simulink model "simulation_basic_sil"  (R2022b)
settings: Solver=ode4  StartTime=0.0  StopTime=3  FixedStep=5e-7  MaxStep=1e-6  RelTol=1e-3
undefined symbols (not defined in the file or in its folder): inverter, motor
libraries: eeGeneralControl x6, mcbcontrolslib x5, SignalEditorBlockLib x2, spsTriangleGeneratorLib x1
settings Model: Creator=Rizwan Sadik  LastModifiedBy=Rizwan Sadik

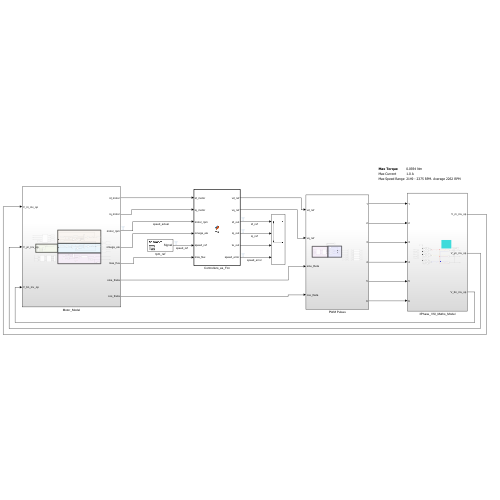
[thumbnail: Simulink's stored preview of the top-level diagram]
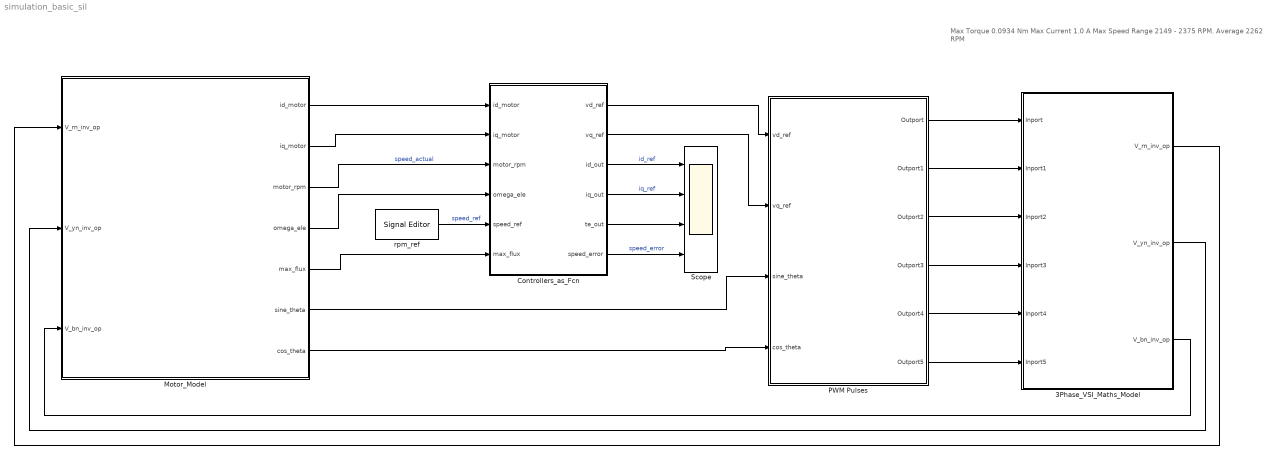
== system simulation_basic_sil ==
  note: Max Torque
      | 0.0934 Nm
      |
      | Max Current
      | 1.0 A
      |
      | Max Speed Range
      | 2149 - 2375 RPM. Average 2262 RPM
  3Phase_VSI_Maths_Model : Subsystem  Description=|
      | Input DC Voltage = Vdc
      | Ouput Phase Voltages = Vrn, Vyn, Vbn
      | 
      | Pole Voltage = Vdc/2
      | Pole Voltages - instantaneous values:
      | Vro = +- Vdc/2
      | Vyo = +- Vdc/2
      | Vbo = +- Vdc/2
      | 
      | Leg 1 o/p is Vr. Switches 1 & 4
      | sw 1 ON (sw 4 OFF) -> Vro = +Vdc/2
      | sw 4 ON (sw 1 OFF) -> Vro = -Vdc/2
      | 
      | Leg 2 o/p is Vy. Switches 3 & 6
      | sw 3 ON (sw 6 OFF) -> Vyo = +Vdc/2
      | sw 6 ON (sw 3 OFF) -> Vyo = -Vdc/2
      | 
      | Leg 3 o/p is Vb. Switches 5 & 2
      | sw 5 ON (sw 2 OFF) -> Vbo = +Vdc/2
      | sw 2 ON (sw 5 OFF) -> Vbo = -Vdc/2
      | 
      | Vrn = (2Vro-Vyo-Vbo)/3
      | Vyn = (2Vyo-Vro-Vbo)/3
      | Vbn =(2Vbo-Vyo-Vro)/3
  Controllers_as_Fcn : MATLAB Function  TreatAsAtomicUnit=on  SystemSampleTime=5e-5
  Motor_Model : Subsystem
  PWM Pulses : Subsystem
  Scope : Scope  NumInputPorts=4
  rpm_ref : SignalEditorBlockLib/Signal Editor  FileName=signal_editor.mat  ActiveScenario=Scenario1  ActiveSignal=Signal  IsBus=off  OutputBusObjectStr=Bus: BusObject  SampleTime=0  ZeroCross=off  OutputAfterFinalValue=Setting to zero  Unit=inherit  PreserveSignalName=on
  wires:
  Motor_Model/3(motor_rpm) -> Controllers_as_Fcn/3(motor_rpm)  "speed_actual"
  Motor_Model/4(omega_ele) -> Controllers_as_Fcn/4(omega_ele)
  PWM Pulses/1(Outport) -> 3Phase_VSI_Maths_Model/1(Inport)
  Motor_Model/5(max_flux) -> Controllers_as_Fcn/6(max_flux)
  PWM Pulses/4(Outport3) -> 3Phase_VSI_Maths_Model/4(Inport3)
  PWM Pulses/5(Outport4) -> 3Phase_VSI_Maths_Model/5(Inport4)
  Motor_Model/6(sine_theta) -> PWM Pulses/3(sine_theta)
  PWM Pulses/3(Outport2) -> 3Phase_VSI_Maths_Model/3(Inport2)
  Motor_Model/2(iq_motor) -> Controllers_as_Fcn/2(iq_motor)
  PWM Pulses/2(Outport1) -> 3Phase_VSI_Maths_Model/2(Inport1)
  PWM Pulses/6(Outport5) -> 3Phase_VSI_Maths_Model/6(Inport5)
  Motor_Model/1(id_motor) -> Controllers_as_Fcn/1(id_motor)
  Motor_Model/7(cos_theta) -> PWM Pulses/4(cos_theta)
  Controllers_as_Fcn/2(vq_ref) -> PWM Pulses/2(vq_ref)
  Controllers_as_Fcn/1(vd_ref) -> PWM Pulses/1(vd_ref)
  3Phase_VSI_Maths_Model/3(V_bn_inv_op) -> Motor_Model/3(V_bn_inv_op)
  3Phase_VSI_Maths_Model/2(V_yn_inv_op) -> Motor_Model/2(V_yn_inv_op)
  3Phase_VSI_Maths_Model/1(V_rn_inv_op) -> Motor_Model/1(V_rn_inv_op)
  rpm_ref/1 -> Controllers_as_Fcn/5(speed_ref)  "speed_ref"
  Controllers_as_Fcn/3(id_out) -> Scope/1  "id_ref"
  Controllers_as_Fcn/4(iq_out) -> Scope/2  "iq_ref"
  Controllers_as_Fcn/5(te_out) -> Scope/3
  Controllers_as_Fcn/6(speed_error) -> Scope/4  "speed_error"

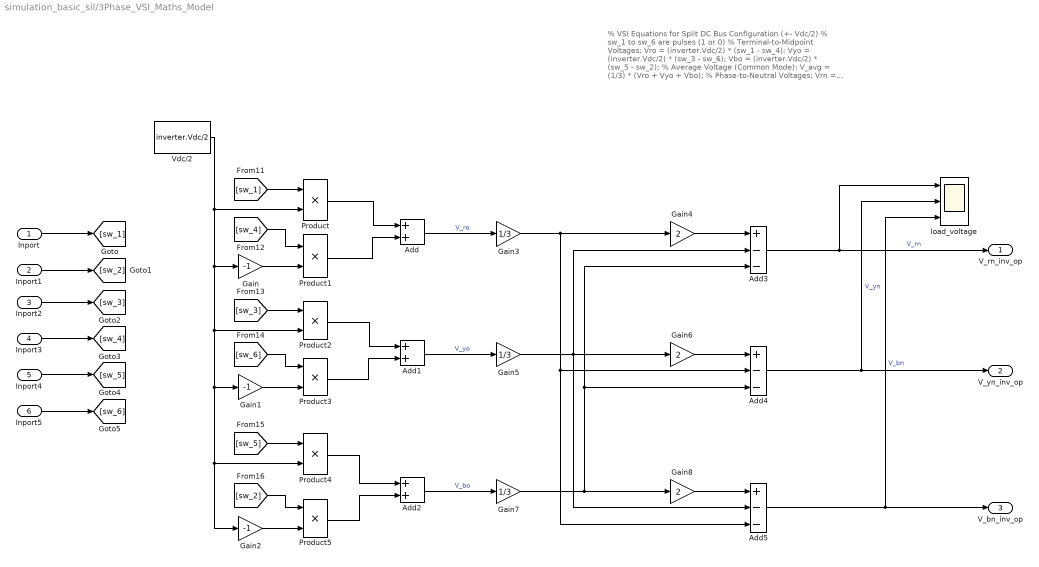
== system simulation_basic_sil/3Phase_VSI_Maths_Model ==
  note: % VSI Equations for Split DC Bus Configuration (+- Vdc/2)
      | % sw_1 to sw_6 are pulses (1 or 0)
      |
      | % Terminal-to-Midpoint Voltages:
      | Vro = (inverter.Vdc/2) * (sw_1 - sw_4);
      | Vyo = (inverter.Vdc/2) * (sw_3 - sw_6);
      | Vbo = (inverter.Vdc/2) * (sw_5 - sw_2);
      |
      | % Average Voltage (Common Mode):
      | V_avg = (1/3) * (Vro + Vyo + Vbo);
      |
      | % Phase-to-Neutral Voltages:
      | Vrn = Vro - V_avg;
      | Vyn = Vyo - V_avg;
      | Vbn = Vbo - V_avg;
  Inport : Inport
  Inport1 : Inport  Port=2
  Inport2 : Inport  Port=3
  Inport3 : Inport  Port=4
  Inport4 : Inport  Port=5
  Inport5 : Inport  Port=6
  Add : Sum
  Add1 : Sum
  Add2 : Sum
  Add3 : Sum  Inputs=+--
  Add4 : Sum  Inputs=+--
  Add5 : Sum  Inputs=+--
  Gain : Gain  Gain=-1
  Gain1 : Gain  Gain=-1
  Gain2 : Gain  Gain=-1
  Gain3 : Gain  Gain=1/3
  Gain4 : Gain  Gain=2
  Gain5 : Gain  Gain=1/3
  Gain6 : Gain  Gain=2
  Gain7 : Gain  Gain=1/3
  Gain8 : Gain  Gain=2
  Product{,1..5} (6 alike) : Product
  Vdc/2 : Constant  Value=inverter.Vdc/2
  load_voltage : Scope  NumInputPorts=3
  V_rn_inv_op : Outport
  V_yn_inv_op : Outport  Port=2
  V_bn_inv_op : Outport  Port=3
  wires:
  Product2/1 -> Add1/1
  Add3/1 -> load_voltage/1, V_rn_inv_op/1  "V_rn"
  Product/1 -> Add/1
  Product4/1 -> Add2/1
  Vdc/2/1 -> Gain2/1, Product4/2, Gain1/1, Product2/2, Gain/1, Product/2
  Gain3/1 -> Add5/3, Add4/2, Gain4/1
  Add4/1 -> load_voltage/2, V_yn_inv_op/1  "V_yn"
  [sw_5] -> Product4/1
  Add/1 -> Gain3/1  "V_ro"
  Gain8/1 -> Add5/1
  Add2/1 -> Gain7/1  "V_bo"
  Gain7/1 -> Gain8/1, Add3/3, Add4/3
  Product5/1 -> Add2/2
  Gain5/1 -> Add5/2, Gain6/1, Add3/2
  [sw_3] -> Product2/1
  Gain4/1 -> Add3/1
  [sw_6] -> Product3/1
  Product3/1 -> Add1/2
  [sw_2] -> Product5/1
  Gain1/1 -> Product3/2
  Gain/1 -> Product1/2
  Product1/1 -> Add/2
  [sw_4] -> Product1/1
  [sw_1] -> Product/1
  Gain2/1 -> Product5/2
  Gain6/1 -> Add4/1
  Add5/1 -> V_bn_inv_op/1, load_voltage/3  "V_bn"
  Inport/1 -> [sw_1]
  Inport1/1 -> [sw_2]
  Inport3/1 -> [sw_4]
  Inport2/1 -> [sw_3]
  Inport5/1 -> [sw_6]
  Inport4/1 -> [sw_5]
  Add1/1 -> Gain5/1  "V_yo"

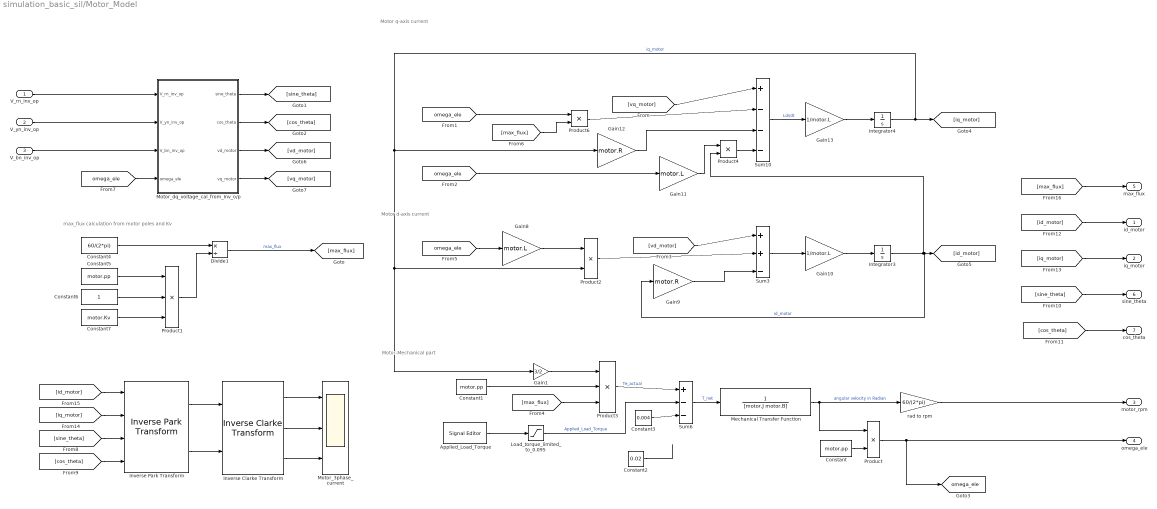
== system simulation_basic_sil/Motor_Model ==
  note: max_flux calculation from motor poles and Kv
  note: Motor-Mechanical part
  note: Motor d-axis current
  note: Motor q-axis current
  V_rn_inv_op : Inport
  V_yn_inv_op : Inport  Port=2
  V_bn_inv_op : Inport  Port=3
  Applied_Load_Torque : SignalEditorBlockLib/Signal Editor  FileName=signal_editor.mat  ActiveScenario=Scenario  ActiveSignal=1  IsBus=off  OutputBusObjectStr=Bus: BusObject  SampleTime=0  ZeroCross=off  OutputAfterFinalValue=Setting to zero  Unit=inherit  PreserveSignalName=on
  Constant : Constant  Value=motor.pp
  Constant1 : Constant  Value=motor.pp
  Constant2 : Constant  Value=0.02
  Constant3 : Constant  Value=0.004
  Constant4 : Constant  Value=60/(2*pi)
  Constant5 : Constant  Value=motor.pp
  Constant6 : Constant
  Constant7 : Constant  Value=motor.Kv
  Divide1 : Product  Inputs=*/
  Gain1 : Gain  Gain=3/2
  Gain10 : Gain  Gain=1/motor.L
  Gain11 : Gain  Gain=motor.L
  Gain12 : Gain  Gain=motor.R
  Gain13 : Gain  Gain=1/motor.L
  Gain8 : Gain  Gain=motor.L
  Gain9 : Gain  Gain=motor.R
  Integrator3 : Integrator
  Integrator4 : Integrator
  Inverse Clarke Transform : mcbcontrolslib/Inverse Clarke Transform
      settings: LibrarySourceBlock=mcbhdllib/Controls/Math Transforms/Inverse Clarke Transform
  Inverse Park Transform : mcbcontrolslib/Inverse Park Transform  AxisAlignment=D-axis
      settings: LibrarySourceBlock=mcblib/Controls/Math Transforms/Inverse Park Transform
  Load_torque_limited_to_0.095 : Saturate  UpperLimit=0.095  LowerLimit=0
  Mechanical Transfer Function : TransferFcn  Denominator=[motor.J motor.B]
  Motor_3phase_current : Scope  NumInputPorts=3
  Motor_dq_voltage_cal_from_Inv_o/p : Subsystem
  Product{,2,4,6} (4 alike) : Product
  Product1 : Product  Inputs=3
  Product3 : Product  Inputs=3
  Sum10 : Sum  Inputs=|+---
  Sum3 : Sum  Inputs=|++-
  Sum6 : Sum  Inputs=+|--
  rad to rpm : Gain  Gain=60/(2*pi)
  id_motor : Outport
  iq_motor : Outport  Port=2
  motor_rpm : Outport  Port=3
  omega_ele : Outport  Port=4
  max_flux : Outport  Port=5
  sine_theta : Outport  Port=6
  cos_theta : Outport  Port=7
  tag scope: omega_ele=global
  wires:
  Product6/1 -> Sum10/2
  Gain12/1 -> Sum10/3
  [max_flux] -> Product6/2
  Gain13/1 -> Integrator4/1
  Gain11/1 -> Product4/1
  Integrator4/1 -> [iq_motor], Gain1/1, Product2/2, Gain12/1  "iq_motor"
  Product4/1 -> Sum10/4
  [omega_ele] -> Gain11/1
  Sum10/1 -> Gain13/1  "Ldi/dt​​"
  [vq_motor] -> Sum10/1
  [omega_ele] -> Product6/1
  Product2/1 -> Sum3/2
  Integrator3/1 -> [id_motor], Gain9/1, Product4/2  "id_motor"
  Gain9/1 -> Sum3/3
  Gain8/1 -> Product2/1
  Sum3/1 -> Gain10/1
  Gain10/1 -> Integrator3/1
  [omega_ele] -> Gain8/1
  [vd_motor] -> Sum3/1
  [max_flux] -> Product3/3
  Constant/1 -> Product/2
  Product/1 -> omega_ele/1, [omega_ele]
  Mechanical Transfer Function/1 -> rad to rpm/1, Product/1  "angular velocity in Radian"
  Sum6/1 -> Mechanical Transfer Function/1  "T_net"
  Constant3/1 -> Sum6/3
  Gain1/1 -> Product3/1
  Product3/1 -> Sum6/1  "Te_actual"
  Load_torque_limited_to_0.095/1 -> Sum6/2  "Applied_Load_Torque"
  Constant1/1 -> Product3/2
  rad to rpm/1 -> motor_rpm/1
  Constant6/1 -> Product1/2
  Product1/1 -> Divide1/2
  Constant5/1 -> Product1/1
  Constant7/1 -> Product1/3
  Constant4/1 -> Divide1/1
  Divide1/1 -> [max_flux]  "max_flux"
  Applied_Load_Torque/1 -> Load_torque_limited_to_0.095/1
  V_rn_inv_op/1 -> Motor_dq_voltage_cal_from_Inv_o/p/1(V_rn_inv_op)
  V_yn_inv_op/1 -> Motor_dq_voltage_cal_from_Inv_o/p/2(V_yn_inv_op)
  V_bn_inv_op/1 -> Motor_dq_voltage_cal_from_Inv_o/p/3(V_bn_inv_op)
  [omega_ele] -> Motor_dq_voltage_cal_from_Inv_o/p/4(omega_ele)
  Motor_dq_voltage_cal_from_Inv_o/p/2(cos_theta) -> [cos_theta]
  Motor_dq_voltage_cal_from_Inv_o/p/3(vd_motor) -> [vd_motor]
  Motor_dq_voltage_cal_from_Inv_o/p/4(vq_motor) -> [vq_motor]
  Inverse Clarke Transform/2 -> Motor_3phase_current/2
  Inverse Clarke Transform/1 -> Motor_3phase_current/1
  Inverse Park Transform/1 -> Inverse Clarke Transform/1
  Inverse Clarke Transform/3 -> Motor_3phase_current/3
  Inverse Park Transform/2 -> Inverse Clarke Transform/2
  Motor_dq_voltage_cal_from_Inv_o/p/1(sine_theta) -> [sine_theta]
  [sine_theta] -> Inverse Park Transform/3
  [cos_theta] -> Inverse Park Transform/4
  [sine_theta] -> sine_theta/1
  [cos_theta] -> cos_theta/1
  [id_motor] -> id_motor/1
  [iq_motor] -> iq_motor/1
  [iq_motor] -> Inverse Park Transform/2
  [id_motor] -> Inverse Park Transform/1
  [max_flux] -> max_flux/1
  Constant2/1 -> ?

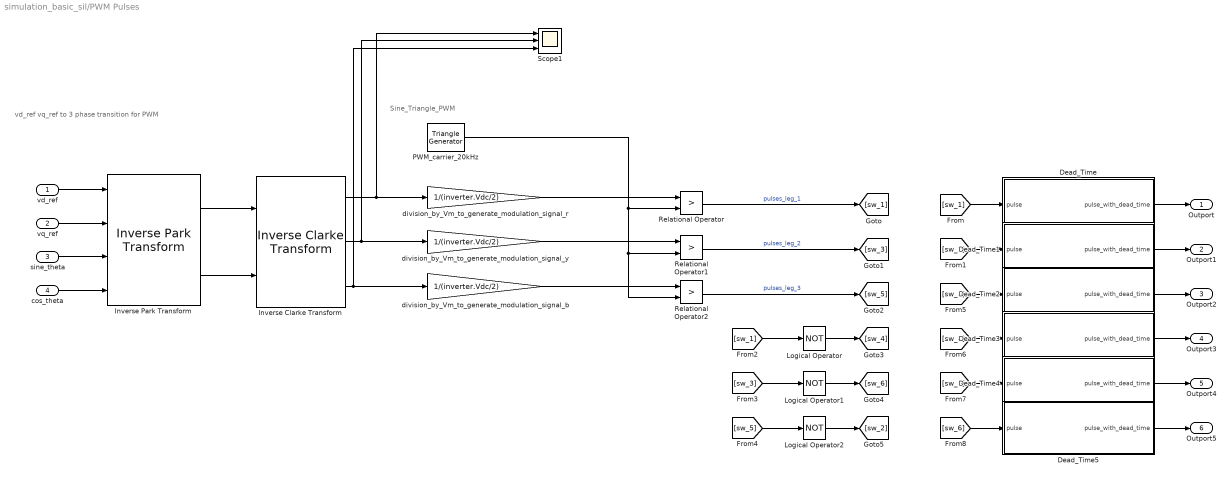
== system simulation_basic_sil/PWM Pulses ==
  note: vd_ref vq_ref to 3 phase transition for PWM
  note: Sine_Triangle_PWM
  vd_ref : Inport
  vq_ref : Inport  Port=2
  sine_theta : Inport  Port=3
  cos_theta : Inport  Port=4
  Dead_Time : Subsystem
  Dead_Time1 : Subsystem
  Dead_Time2 : Subsystem
  Dead_Time3 : Subsystem
  Dead_Time4 : Subsystem
  Dead_Time5 : Subsystem
  Inverse Clarke Transform : mcbcontrolslib/Inverse Clarke Transform
      settings: LibrarySourceBlock=mcbhdllib/Controls/Math Transforms/Inverse Clarke Transform
  Inverse Park Transform : mcbcontrolslib/Inverse Park Transform  AxisAlignment=D-axis
      settings: LibrarySourceBlock=mcblib/Controls/Math Transforms/Inverse Park Transform
  Logical Operator : Logic  Operator=NOT  AllPortsSameDT=off  OutDataTypeStr=boolean
  Logical Operator1 : Logic  Operator=NOT  AllPortsSameDT=off  OutDataTypeStr=boolean
  Logical Operator2 : Logic  Operator=NOT  AllPortsSameDT=off  OutDataTypeStr=boolean
  PWM_carrier_20kHz : spsTriangleGeneratorLib/Triangle Generator  Freq=20000  Phase=0  Ts=0
  Relational Operator : RelationalOperator  Operator=>  OutDataTypeStr=boolean  RndMeth=Simplest  InputSameDT=off
  Relational Operator1 : RelationalOperator  Operator=>  OutDataTypeStr=boolean  RndMeth=Simplest  InputSameDT=off
  Relational Operator2 : RelationalOperator  Operator=>  OutDataTypeStr=boolean  RndMeth=Simplest  InputSameDT=off
  Scope1 : Scope  NumInputPorts=3
  division_by_Vm_to_generate_modulation_signal_b : Gain  Gain=1/(inverter.Vdc/2)
  division_by_Vm_to_generate_modulation_signal_r : Gain  Gain=1/(inverter.Vdc/2)
  division_by_Vm_to_generate_modulation_signal_y : Gain  Gain=1/(inverter.Vdc/2)
  Outport : Outport
  Outport1 : Outport  Port=2
  Outport2 : Outport  Port=3
  Outport3 : Outport  Port=4
  Outport4 : Outport  Port=5
  Outport5 : Outport  Port=6
  wires:
  [sw_3] -> Logical Operator1/1
  Logical Operator2/1 -> [sw_2]
  cos_theta/1 -> Inverse Park Transform/4
  sine_theta/1 -> Inverse Park Transform/3
  [sw_5] -> Logical Operator2/1
  Inverse Park Transform/2 -> Inverse Clarke Transform/2
  Inverse Park Transform/1 -> Inverse Clarke Transform/1
  Logical Operator/1 -> [sw_4]
  Logical Operator1/1 -> [sw_6]
  [sw_1] -> Logical Operator/1
  vd_ref/1 -> Inverse Park Transform/1
  vq_ref/1 -> Inverse Park Transform/2
  [sw_1] -> Dead_Time/1(pulse)
  [sw_6] -> Dead_Time5/1(pulse)
  [sw_2] -> Dead_Time1/1(pulse)
  [sw_3] -> Dead_Time2/1(pulse)
  [sw_4] -> Dead_Time3/1(pulse)
  [sw_5] -> Dead_Time4/1(pulse)
  Relational Operator2/1 -> [sw_5]  "pulses_leg_3"
  Relational Operator1/1 -> [sw_3]  "pulses_leg_2"
  Relational Operator/1 -> [sw_1]  "pulses_leg_1"
  PWM_carrier_20kHz/1 -> Relational Operator2/2, Relational Operator1/2, Relational Operator/2
  division_by_Vm_to_generate_modulation_signal_y/1 -> Relational Operator1/1
  division_by_Vm_to_generate_modulation_signal_b/1 -> Relational Operator2/1
  Inverse Clarke Transform/3 -> Scope1/3, division_by_Vm_to_generate_modulation_signal_b/1
  Inverse Clarke Transform/2 -> Scope1/2, division_by_Vm_to_generate_modulation_signal_y/1
  division_by_Vm_to_generate_modulation_signal_r/1 -> Relational Operator/1
  Inverse Clarke Transform/1 -> Scope1/1, division_by_Vm_to_generate_modulation_signal_r/1
  Dead_Time/1(pulse_with_dead_time) -> Outport/1
  Dead_Time1/1(pulse_with_dead_time) -> Outport1/1
  Dead_Time2/1(pulse_with_dead_time) -> Outport2/1
  Dead_Time3/1(pulse_with_dead_time) -> Outport3/1
  Dead_Time4/1(pulse_with_dead_time) -> Outport4/1
  Dead_Time5/1(pulse_with_dead_time) -> Outport5/1

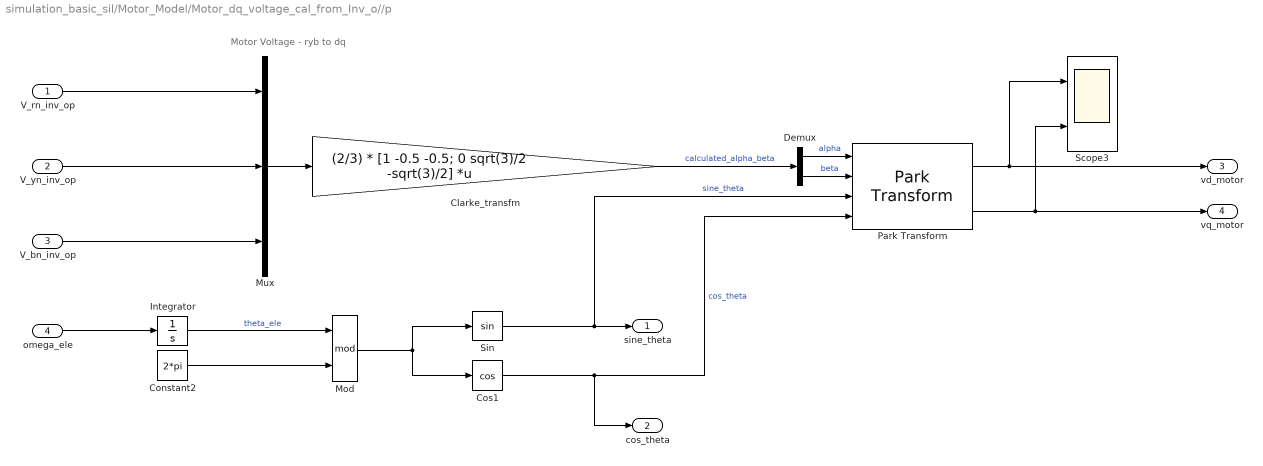
== system simulation_basic_sil/Motor_Model/Motor_dq_voltage_cal_from_Inv_o//p ==
  note: Motor Voltage - ryb to dq
  V_rn_inv_op : Inport
  V_yn_inv_op : Inport  Port=2
  V_bn_inv_op : Inport  Port=3
  omega_ele : Inport  Port=4
  Clarke_transfm : Gain  Gain=(2/3) * [1 -0.5 -0.5; 0 sqrt(3)/2 -sqrt(3)/2]  Multiplication=Matrix(K*u)
  Constant2 : Constant  Value=2*pi
  Cos1 : Trigonometry  Operator=cos
  Demux : Demux  Outputs=2
  Integrator : Integrator
  Mod : Math  Operator=mod
  Mux : Mux  Inputs=3
  Park Transform : mcbcontrolslib/Park Transform  AxisAlignment=D-axis
      settings: LibrarySourceBlock=mcbhdllib/Controls/Math Transforms/Park Transform
  Scope3 : Scope  NumInputPorts=2
  Sin : Trigonometry
  sine_theta : Outport
  cos_theta : Outport  Port=2
  vd_motor : Outport  Port=3
  vq_motor : Outport  Port=4
  wires:
  Sin/1 -> sine_theta/1, Park Transform/3  "sine_theta"
  Constant2/1 -> Mod/2
  Cos1/1 -> cos_theta/1, Park Transform/4  "cos_theta"
  Mod/1 -> Cos1/1, Sin/1
  Demux/1 -> Park Transform/1  "alpha"
  Park Transform/2 -> Scope3/2, vq_motor/1
  Clarke_transfm/1 -> Demux/1  "calculated_alpha_beta"
  Integrator/1 -> Mod/1  "theta_ele"
  Demux/2 -> Park Transform/2  "beta"
  Mux/1 -> Clarke_transfm/1
  Park Transform/1 -> vd_motor/1, Scope3/1
  V_bn_inv_op/1 -> Mux/3
  omega_ele/1 -> Integrator/1
  V_rn_inv_op/1 -> Mux/1
  V_yn_inv_op/1 -> Mux/2

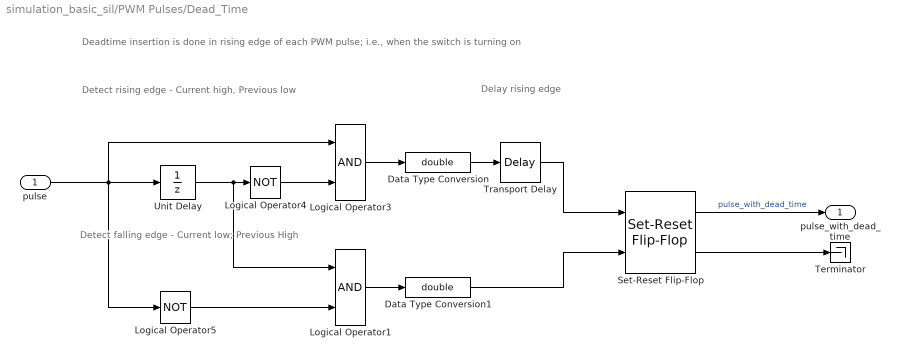
== system simulation_basic_sil/PWM Pulses/Dead_Time ==
  note: Deadtime insertion is done in rising edge of each PWM pulse; i.e., when the switch is turning on
  note: Delay rising edge
  note: Detect falling edge - Current low; Previous High
  note: Detect rising edge - Current high, Previous low
  pulse : Inport
  Data Type Conversion : DataTypeConversion  OutDataTypeStr=double  SaturateOnIntegerOverflow=off  RndMeth=Floor
  Data Type Conversion1 : DataTypeConversion  OutDataTypeStr=double  SaturateOnIntegerOverflow=off  RndMeth=Floor
  Logical Operator1 : Logic  AllPortsSameDT=off  OutDataTypeStr=boolean
  Logical Operator3 : Logic  AllPortsSameDT=off  OutDataTypeStr=boolean
  Logical Operator4 : Logic  Operator=NOT  AllPortsSameDT=off  OutDataTypeStr=boolean
  Logical Operator5 : Logic  Operator=NOT  AllPortsSameDT=off  OutDataTypeStr=boolean
  Set-Reset Flip-Flop : eeGeneralControl/Set-Reset Flip-Flop  LabelModeActiveChoice=Discrete  UndefState=Set  Q0=0  Ts=-1
      settings: LibrarySourceBlock=ee_sl_lib/General Control/Set-Reset Flip-Flop
  Terminator : Terminator
  Transport Delay : TransportDelay  DelayTime=2e-6
  Unit Delay : UnitDelay  SampleTime=-1  HasFrameUpgradeWarning=on
  pulse_with_dead_time : Outport
  wires:
  Unit Delay/1 -> Logical Operator1/1, Logical Operator4/1
  pulse/1 -> Logical Operator5/1, Logical Operator3/1, Unit Delay/1
  Logical Operator5/1 -> Logical Operator1/2
  Logical Operator4/1 -> Logical Operator3/2
  Transport Delay/1 -> Set-Reset Flip-Flop/1
  Data Type Conversion/1 -> Transport Delay/1
  Logical Operator3/1 -> Data Type Conversion/1
  Data Type Conversion1/1 -> Set-Reset Flip-Flop/2
  Logical Operator1/1 -> Data Type Conversion1/1
  Set-Reset Flip-Flop/1 -> pulse_with_dead_time/1  "pulse_with_dead_time"
  Set-Reset Flip-Flop/2 -> Terminator/1

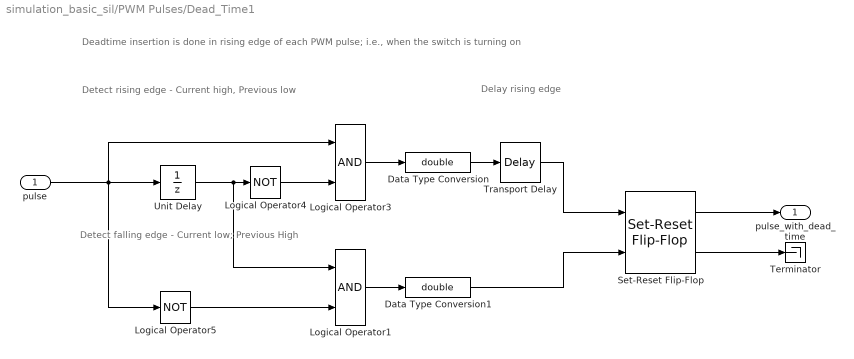
== system simulation_basic_sil/PWM Pulses/Dead_Time1 ==
  note: Detect rising edge - Current high, Previous low
  note: Detect falling edge - Current low; Previous High
  note: Delay rising edge
  note: Deadtime insertion is done in rising edge of each PWM pulse; i.e., when the switch is turning on
  pulse : Inport
  Data Type Conversion : DataTypeConversion  OutDataTypeStr=double  SaturateOnIntegerOverflow=off  RndMeth=Floor
  Data Type Conversion1 : DataTypeConversion  OutDataTypeStr=double  SaturateOnIntegerOverflow=off  RndMeth=Floor
  Logical Operator1 : Logic  AllPortsSameDT=off  OutDataTypeStr=boolean
  Logical Operator3 : Logic  AllPortsSameDT=off  OutDataTypeStr=boolean
  Logical Operator4 : Logic  Operator=NOT  AllPortsSameDT=off  OutDataTypeStr=boolean
  Logical Operator5 : Logic  Operator=NOT  AllPortsSameDT=off  OutDataTypeStr=boolean
  Set-Reset Flip-Flop : eeGeneralControl/Set-Reset Flip-Flop  LabelModeActiveChoice=Discrete  UndefState=Set  Q0=0  Ts=-1
      settings: LibrarySourceBlock=ee_sl_lib/General Control/Set-Reset Flip-Flop
  Terminator : Terminator
  Transport Delay : TransportDelay  DelayTime=2e-6
  Unit Delay : UnitDelay  SampleTime=-1  HasFrameUpgradeWarning=on
  pulse_with_dead_time : Outport
  wires:
  Set-Reset Flip-Flop/2 -> Terminator/1
  Set-Reset Flip-Flop/1 -> pulse_with_dead_time/1
  Logical Operator1/1 -> Data Type Conversion1/1
  Data Type Conversion1/1 -> Set-Reset Flip-Flop/2
  Logical Operator3/1 -> Data Type Conversion/1
  Data Type Conversion/1 -> Transport Delay/1
  Transport Delay/1 -> Set-Reset Flip-Flop/1
  Logical Operator4/1 -> Logical Operator3/2
  Logical Operator5/1 -> Logical Operator1/2
  pulse/1 -> Unit Delay/1, Logical Operator3/1, Logical Operator5/1
  Unit Delay/1 -> Logical Operator4/1, Logical Operator1/1

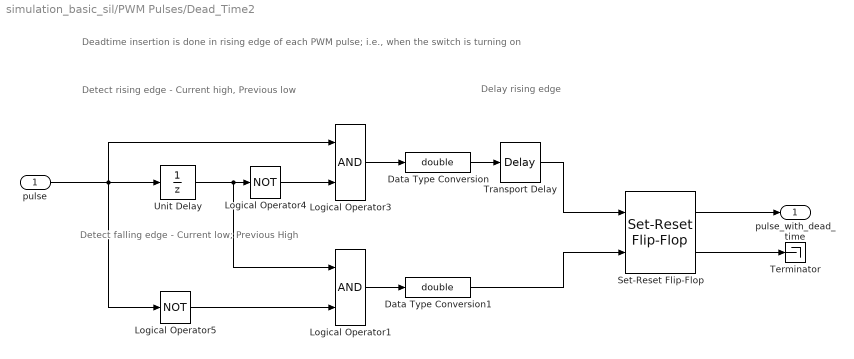
== system simulation_basic_sil/PWM Pulses/Dead_Time2 ==
  note: Deadtime insertion is done in rising edge of each PWM pulse; i.e., when the switch is turning on
  note: Delay rising edge
  note: Detect falling edge - Current low; Previous High
  note: Detect rising edge - Current high, Previous low
  pulse : Inport
  Data Type Conversion : DataTypeConversion  OutDataTypeStr=double  SaturateOnIntegerOverflow=off  RndMeth=Floor
  Data Type Conversion1 : DataTypeConversion  OutDataTypeStr=double  SaturateOnIntegerOverflow=off  RndMeth=Floor
  Logical Operator1 : Logic  AllPortsSameDT=off  OutDataTypeStr=boolean
  Logical Operator3 : Logic  AllPortsSameDT=off  OutDataTypeStr=boolean
  Logical Operator4 : Logic  Operator=NOT  AllPortsSameDT=off  OutDataTypeStr=boolean
  Logical Operator5 : Logic  Operator=NOT  AllPortsSameDT=off  OutDataTypeStr=boolean
  Set-Reset Flip-Flop : eeGeneralControl/Set-Reset Flip-Flop  LabelModeActiveChoice=Discrete  UndefState=Set  Q0=0  Ts=-1
      settings: LibrarySourceBlock=ee_sl_lib/General Control/Set-Reset Flip-Flop
  Terminator : Terminator
  Transport Delay : TransportDelay  DelayTime=2e-6
  Unit Delay : UnitDelay  SampleTime=-1  HasFrameUpgradeWarning=on
  pulse_with_dead_time : Outport
  wires:
  Unit Delay/1 -> Logical Operator1/1, Logical Operator4/1
  pulse/1 -> Logical Operator5/1, Logical Operator3/1, Unit Delay/1
  Logical Operator5/1 -> Logical Operator1/2
  Logical Operator4/1 -> Logical Operator3/2
  Transport Delay/1 -> Set-Reset Flip-Flop/1
  Data Type Conversion/1 -> Transport Delay/1
  Logical Operator3/1 -> Data Type Conversion/1
  Data Type Conversion1/1 -> Set-Reset Flip-Flop/2
  Logical Operator1/1 -> Data Type Conversion1/1
  Set-Reset Flip-Flop/1 -> pulse_with_dead_time/1
  Set-Reset Flip-Flop/2 -> Terminator/1

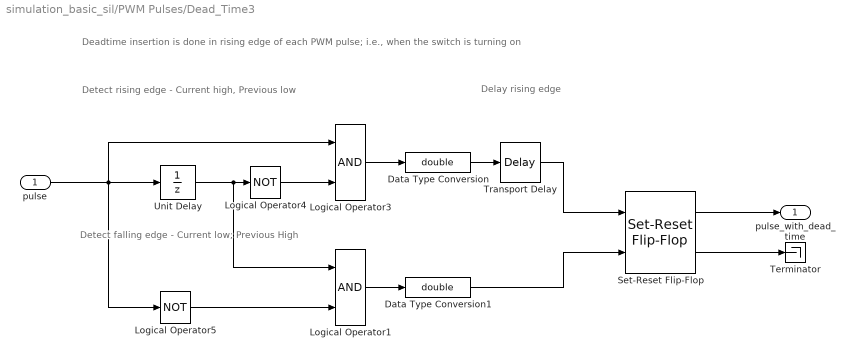
== system simulation_basic_sil/PWM Pulses/Dead_Time3 ==
  note: Detect rising edge - Current high, Previous low
  note: Detect falling edge - Current low; Previous High
  note: Delay rising edge
  note: Deadtime insertion is done in rising edge of each PWM pulse; i.e., when the switch is turning on
  pulse : Inport
  Data Type Conversion : DataTypeConversion  OutDataTypeStr=double  SaturateOnIntegerOverflow=off  RndMeth=Floor
  Data Type Conversion1 : DataTypeConversion  OutDataTypeStr=double  SaturateOnIntegerOverflow=off  RndMeth=Floor
  Logical Operator1 : Logic  AllPortsSameDT=off  OutDataTypeStr=boolean
  Logical Operator3 : Logic  AllPortsSameDT=off  OutDataTypeStr=boolean
  Logical Operator4 : Logic  Operator=NOT  AllPortsSameDT=off  OutDataTypeStr=boolean
  Logical Operator5 : Logic  Operator=NOT  AllPortsSameDT=off  OutDataTypeStr=boolean
  Set-Reset Flip-Flop : eeGeneralControl/Set-Reset Flip-Flop  LabelModeActiveChoice=Discrete  UndefState=Set  Q0=0  Ts=-1
      settings: LibrarySourceBlock=ee_sl_lib/General Control/Set-Reset Flip-Flop
  Terminator : Terminator
  Transport Delay : TransportDelay  DelayTime=2e-6
  Unit Delay : UnitDelay  SampleTime=-1  HasFrameUpgradeWarning=on
  pulse_with_dead_time : Outport
  wires:
  Set-Reset Flip-Flop/2 -> Terminator/1
  Set-Reset Flip-Flop/1 -> pulse_with_dead_time/1
  Logical Operator1/1 -> Data Type Conversion1/1
  Data Type Conversion1/1 -> Set-Reset Flip-Flop/2
  Logical Operator3/1 -> Data Type Conversion/1
  Data Type Conversion/1 -> Transport Delay/1
  Transport Delay/1 -> Set-Reset Flip-Flop/1
  Logical Operator4/1 -> Logical Operator3/2
  Logical Operator5/1 -> Logical Operator1/2
  pulse/1 -> Unit Delay/1, Logical Operator3/1, Logical Operator5/1
  Unit Delay/1 -> Logical Operator4/1, Logical Operator1/1

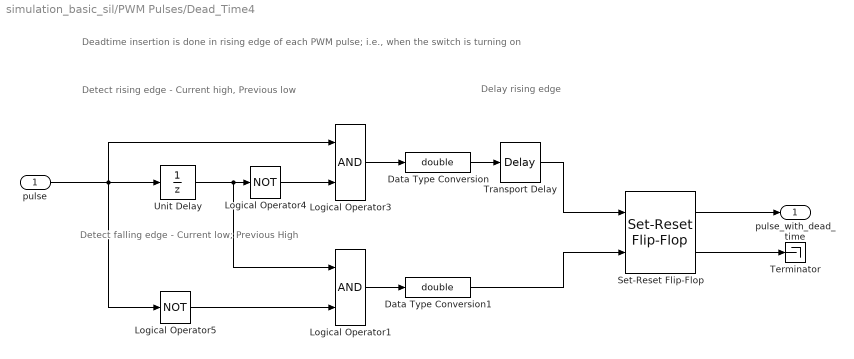
== system simulation_basic_sil/PWM Pulses/Dead_Time4 ==
  note: Deadtime insertion is done in rising edge of each PWM pulse; i.e., when the switch is turning on
  note: Delay rising edge
  note: Detect falling edge - Current low; Previous High
  note: Detect rising edge - Current high, Previous low
  pulse : Inport
  Data Type Conversion : DataTypeConversion  OutDataTypeStr=double  SaturateOnIntegerOverflow=off  RndMeth=Floor
  Data Type Conversion1 : DataTypeConversion  OutDataTypeStr=double  SaturateOnIntegerOverflow=off  RndMeth=Floor
  Logical Operator1 : Logic  AllPortsSameDT=off  OutDataTypeStr=boolean
  Logical Operator3 : Logic  AllPortsSameDT=off  OutDataTypeStr=boolean
  Logical Operator4 : Logic  Operator=NOT  AllPortsSameDT=off  OutDataTypeStr=boolean
  Logical Operator5 : Logic  Operator=NOT  AllPortsSameDT=off  OutDataTypeStr=boolean
  Set-Reset Flip-Flop : eeGeneralControl/Set-Reset Flip-Flop  LabelModeActiveChoice=Discrete  UndefState=Set  Q0=0  Ts=-1
      settings: LibrarySourceBlock=ee_sl_lib/General Control/Set-Reset Flip-Flop
  Terminator : Terminator
  Transport Delay : TransportDelay  DelayTime=2e-6
  Unit Delay : UnitDelay  SampleTime=-1  HasFrameUpgradeWarning=on
  pulse_with_dead_time : Outport
  wires:
  Unit Delay/1 -> Logical Operator1/1, Logical Operator4/1
  pulse/1 -> Logical Operator5/1, Logical Operator3/1, Unit Delay/1
  Logical Operator5/1 -> Logical Operator1/2
  Logical Operator4/1 -> Logical Operator3/2
  Transport Delay/1 -> Set-Reset Flip-Flop/1
  Data Type Conversion/1 -> Transport Delay/1
  Logical Operator3/1 -> Data Type Conversion/1
  Data Type Conversion1/1 -> Set-Reset Flip-Flop/2
  Logical Operator1/1 -> Data Type Conversion1/1
  Set-Reset Flip-Flop/1 -> pulse_with_dead_time/1
  Set-Reset Flip-Flop/2 -> Terminator/1

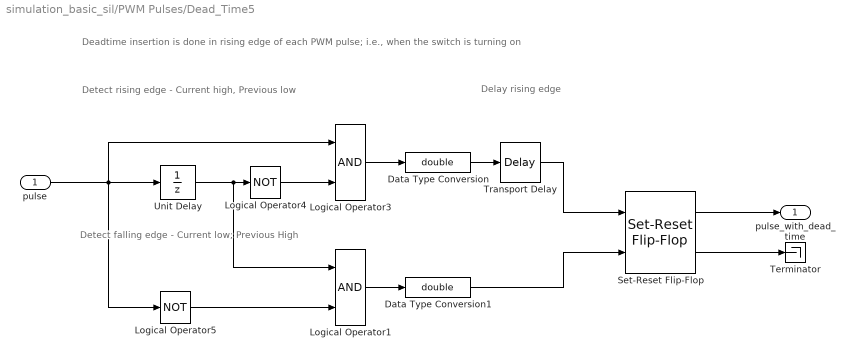
== system simulation_basic_sil/PWM Pulses/Dead_Time5 ==
  note: Detect rising edge - Current high, Previous low
  note: Detect falling edge - Current low; Previous High
  note: Delay rising edge
  note: Deadtime insertion is done in rising edge of each PWM pulse; i.e., when the switch is turning on
  pulse : Inport
  Data Type Conversion : DataTypeConversion  OutDataTypeStr=double  SaturateOnIntegerOverflow=off  RndMeth=Floor
  Data Type Conversion1 : DataTypeConversion  OutDataTypeStr=double  SaturateOnIntegerOverflow=off  RndMeth=Floor
  Logical Operator1 : Logic  AllPortsSameDT=off  OutDataTypeStr=boolean
  Logical Operator3 : Logic  AllPortsSameDT=off  OutDataTypeStr=boolean
  Logical Operator4 : Logic  Operator=NOT  AllPortsSameDT=off  OutDataTypeStr=boolean
  Logical Operator5 : Logic  Operator=NOT  AllPortsSameDT=off  OutDataTypeStr=boolean
  Set-Reset Flip-Flop : eeGeneralControl/Set-Reset Flip-Flop  LabelModeActiveChoice=Discrete  UndefState=Set  Q0=0  Ts=-1
      settings: LibrarySourceBlock=ee_sl_lib/General Control/Set-Reset Flip-Flop
  Terminator : Terminator
  Transport Delay : TransportDelay  DelayTime=2e-6
  Unit Delay : UnitDelay  SampleTime=-1  HasFrameUpgradeWarning=on
  pulse_with_dead_time : Outport
  wires:
  Set-Reset Flip-Flop/2 -> Terminator/1
  Set-Reset Flip-Flop/1 -> pulse_with_dead_time/1
  Logical Operator1/1 -> Data Type Conversion1/1
  Data Type Conversion1/1 -> Set-Reset Flip-Flop/2
  Logical Operator3/1 -> Data Type Conversion/1
  Data Type Conversion/1 -> Transport Delay/1
  Transport Delay/1 -> Set-Reset Flip-Flop/1
  Logical Operator4/1 -> Logical Operator3/2
  Logical Operator5/1 -> Logical Operator1/2
  pulse/1 -> Unit Delay/1, Logical Operator3/1, Logical Operator5/1
  Unit Delay/1 -> Logical Operator4/1, Logical Operator1/1

== matlab function simulation_basic_sil/Controllers_as_Fcn ==
  settings: updateMethod=DISCRETE
  data: id_motor input; iq_motor input; motor_rpm input; omega_ele input; speed_ref input; vd_ref output; vq_ref output; id_out output; iq_out output; te_out output; speed_error output; max_flux input
function [vd_ref, vq_ref, id_out, iq_out, te_out, speed_error] = fcn(id_motor, iq_motor, motor_rpm, omega_ele, speed_ref, max_flux)
    [vd_ref, vq_ref, id_out, iq_out, te_out, speed_error] = foc_algorithm_sil_16_04_26(id_motor, iq_motor, motor_rpm, omega_ele, speed_ref, max_flux);
end
